simulink model "CARV_bf_simu"  (R2018a)
settings: Solver=ode5  StartTime=0.0  StopTime=10  FixedStep=Te  RelTol=1e-3
values from neighbouring files (symbols this model uses):
  R = 0    [RST_eleve.m]
  S = 1    [RST_eleve.m]
  Te = 1/800    (= 0.00125)    [RST_eleve.m]
  wd = 450    [RST_eleve.m]
CloseFcn:
  | rtwprivate ssgencode ModelCloseRequest Poulies_bf
settings Model: ExtModeTrigDuration=60000  Creator=drey  LastModifiedBy=khennouh
settings DataIOCC: SaveFormat=Array  SignalLoggingSaveFormat=ModelDataLogs
settings OptimizationCC: BlockReduction=off  BooleanDataType=off  ExpressionDepthLimit=2147483647  InitFltsAndDblsToZero=on  LifeSpan=inf
settings DebuggingCC: SaveWithParameterizedLinksMsg=none  UnderspecifiedInitializationDetection=Classic  MergeDetectMultiDrivingBlocksExec=none  SignalResolutionControl=TryResolveAllWithWarning  MultiTaskDSMMsg=warning  MultiTaskCondExecSysMsg=none  FcnCallInpInsideContextMsg=warning  StateNameClashWarn=warning  SFUnexpectedBacktrackingDiag=warning  SFNoUnconditionalDefaultTransitionDiag=warning  SFExecutionAtInitializationDiag=none
settings HardwareCC: ProdBitPerPointer=32  ProdBitPerSizeT=32  ProdBitPerPtrDiffT=32  ProdLargestAtomicFloat=None  ProdIntDivRoundTo=Undefined  ProdEndianess=Unspecified  ProdWordSize=32  ProdHWDeviceType=32-bit Generic
settings ModelReferenceCC: PropagateSignalLabelsOutOfModel=off
settings RTWCC: SystemTargetFile=rtwin.tlc  TemplateMakefile=rtwin.tmf  Description=Real-Time Windows Target
settings CodeAppCC: StateflowObjectComments=on
settings TargetCC: TargetFcnLib=ansi_tfl_tmw.mat  ModelReferenceCompliant=off  CompOptLevelCompliant=off  GeneratePreprocessorConditionals=Use local settings
settings ConfigComp: CovMetricSettings=dw  CovHtmlReporting=on  CovSaveCumulativeToWorkspaceVar=on  CovSaveSingleToWorkspaceVar=on  CovExternalEMLEnable=off

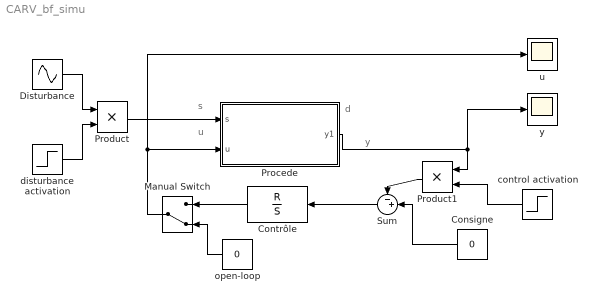
== system CARV_bf_simu ==
  note: d
  note: y
  note: s
  note: u
  Consigne : Constant  Value=0
  Contrôle : DiscreteFilter  Numerator=R  Denominator=S  SampleTime=Te
  Disturbance : Sin  Amplitude=0.02  Frequency=wd  SampleTime=Te
  Manual Switch : ManualSwitch  CurrentSetting=0
  Procede : Subsystem
      mask Display: disp('Procédé Simulé')
  Product : Product  RndMeth=Zero
  Product1 : Product  RndMeth=Zero
  Sum : Sum  Inputs=-+|
  control activation : Step  Time=4  SampleTime=0
  disturbance activation : Step  Time=2  SampleTime=0
  open-loop : Constant  Value=0
  u : Scope
  y : Scope
  wires:
  Procede/1(y1) -> Product1/1, y/1
  Consigne/1 -> Sum/2
  Sum/1 -> Contrôle/1
  Contrôle/1 -> Manual Switch/1
  Manual Switch/1 -> Procede/2(u), u/1
  open-loop/1 -> Manual Switch/2
  Product/1 -> Procede/1(s)
  disturbance activation/1 -> Product/2
  control activation/1 -> Product1/2
  Disturbance/1 -> Product/1
  Product1/1 -> Sum/1

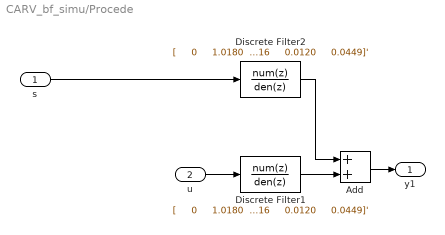
== system CARV_bf_simu/Procede ==
  s : Inport
  u : Inport  Port=2
  Add : Sum
  Discrete Filter1 : DiscreteFilter  Numerator=|  Denominator=|  SampleTime=Te
      Numerator=|
      | [     0
      |     1.0180
      |    -2.1169
      |     0.6843
      |    -0.3008
      |     2.9943
      |    -3.0203
      |     0.8812
      |    -1.5539
      |     2.2356
      |    -0.7953
      |     0.6724
      |    -1.0735
      |     0.1364
      |     0.2454]'
      Denominator=|
      | [1.0000
      |    -1.7389
      |     1.0408
      |    -0.7931
      |     2.5618
      |    -2.8601
      |     1.7853
      |    -1.7239
      |     2.0897
      |    -1.2512
      |     1.0092
      |    -1.0000
      |     0.5016
      |     0.0120
      |     0.0449]'
  Discrete Filter2 : DiscreteFilter  Numerator=|  Denominator=|  SampleTime=Te
      Numerator=|
      | [     0
      |     1.0180
      |    -2.1169
      |     0.6843
      |    -0.3008
      |     2.9943
      |    -3.0203
      |     0.8812
      |    -1.5539
      |     2.2356
      |    -0.7953
      |     0.6724
      |    -1.0735
      |     0.1364
      |     0.2454]'
      Denominator=|
      | [1.0000
      |    -1.7389
      |     1.0408
      |    -0.7931
      |     2.5618
      |    -2.8601
      |     1.7853
      |    -1.7239
      |     2.0897
      |    -1.2512
      |     1.0092
      |    -1.0000
      |     0.5016
      |     0.0120
      |     0.0449]'
  y1 : Outport
  wires:
  s/1 -> Discrete Filter2/1
  u/1 -> Discrete Filter1/1
  Discrete Filter2/1 -> Add/1
  Discrete Filter1/1 -> Add/2
  Add/1 -> y1/1
